simulink model "cart_pendulam"  (R2019a)
settings: Solver=VariableStepAuto  StartTime=0.0  StopTime=inf  FixedStep=0.01  MaxStep=0.05  MinStep=0.001  RelTol=1e-3
undefined symbols (not defined in the file): sigbuilder_block
settings Model: Creator=HPP  LastModifiedBy=vardhah
settings SolverCC: InitialStep=0.01
settings DebuggingCC: UnderSpecifiedDimensionMsg=warning

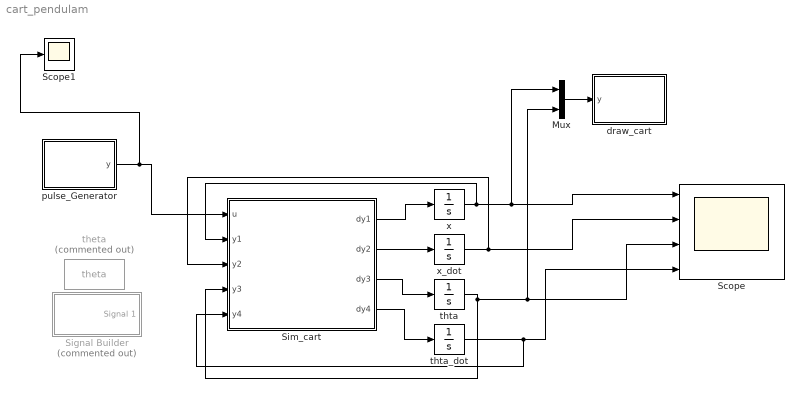
== system cart_pendulam ==
  Mux : Mux  Inputs=2
  Scope : Scope  NumInputPorts=4
  Scope1 : Scope
  Signal Builder : Subsystem  Tag=STV Subsys  Commented=on  LoadFcn=sigbuilder_block('load');  StartFcn=sigbuilder_block('start');  StopFcn=sigbuilder_block('stop');  ClipboardFcn=sigbuilder_block('clipboard');  mask(Sigbuilder block){tuvar=[0:10]}
      mask help: Simulink:masks:SigbuilderBlock_MD
      mask init:
      | if ~strcmp(get_param(bdroot(gcbh),'SimulationStatus'),'stopped') tuvar = sigbuilder_block('maskInit'); end
      settings: CopyFcn=sigbuilder_block('copy');  DeleteFcn=sigbuilder_block('delete');  ModelCloseFcn=sigbuilder_block('modelClose');  PreSaveFcn=sigbuilder_block('preSave');  PauseFcn=sigbuilder_block('pause');  ContinueFcn=sigbuilder_block('continue');  NameChangeFcn=sigbuilder_block('namechange');  OpenFcn=sigbuilder_block('open',[437.6 199.2 550.4 400 ]);  CloseFcn=sigbuilder_block('close');
      mask Display: plot(0, 0, 100, 100,[2, 2, 32, 32, 2], [68, 8, 8, 68, 68],[32, 2], [38, 38], [32, 19, 2],[53, 60, 44], [32, 17, 17, 2],[16, 16, 31, 31]);txt = getActiveGroup(gcbh);text(2, 100, txt,'verticalAlignment', 'top');
  Sim_cart : MATLAB Function  TreatAsAtomicUnit=on
  draw_cart : MATLAB Function  TreatAsAtomicUnit=on
  pulse_Generator : MATLAB Function  TreatAsAtomicUnit=on
  theta : ToWorkspace  Commented=on  VariableName=theta  SaveFormat=Timeseries  SampleTime=-1
  thta : Integrator
  thta_dot : Integrator
  x : Integrator
  x_dot : Integrator
  wires:
  Sim_cart/1(dy1) -> x/1
  Sim_cart/2(dy2) -> x_dot/1
  Sim_cart/3(dy3) -> thta/1
  Sim_cart/4(dy4) -> thta_dot/1
  x/1 -> Sim_cart/2(y1), Mux/1, Scope/1
  x_dot/1 -> Sim_cart/3(y2), Scope/2
  thta_dot/1 -> Sim_cart/5(y4), Scope/4
  pulse_Generator/1(y) -> Scope1/1, Sim_cart/1(u)
  thta/1 -> Sim_cart/4(y3), Mux/2, Scope/3
  Mux/1 -> draw_cart/1(y)

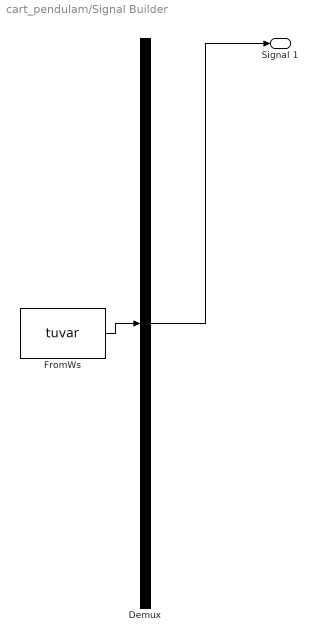
== system cart_pendulam/Signal Builder ==
  Demux : Demux  Tag=STV Demux  Outputs=1
  FromWs : FromWorkspace  Tag=STV FromWs  VariableName=tuvar  SampleTime=0
      SigBuilderData=|
      | common.afterFinalStr = 'Extrapolate'
      | common.sampleTime = 0
      | dataSet.timeRange = [0 10]
      | dataSet.name = 'Group 1'
      | sbobj.Groups.Name = 'Group 1'
      | sbobj.Groups.Signals.Name = 'Signal 1'
      | sbobj.Groups.Signals.XData = [0 4 4 6 6 10]
      | sbobj.Groups.Signals.YData = [0 0 1 1 0 0]
  Signal 1 : Outport  Tag=STV Outport
  wires:
  Demux/1 -> Signal 1/1
  FromWs/1 -> Demux/1

== matlab function cart_pendulam/draw_cart ==
  data: y input
function drawcartpend(y)
x = y(1);
th = y(2);

m = 1;
M = 5;
L = 2;
% kinematics
% x = 3;        % cart position
% th = 3*pi/2;   % pendulum angle

% dimensions
% L = 2;  % pendulum length
W = 1*sqrt(M/5);  % cart width
H = .5*sqrt(M/5); % cart height
wr = .2; % wheel radius
mr = .3*sqrt(m); % mass radius

% positions
% y = wr/2; % cart vertical position
y = wr/2+H/2; % cart vertical position
w1x = x-.9*W/2;
w1y = 0;
w2x = x+.9*W/2-wr;
w2y = 0;

px = x + L*sin(th);
py = y - L*cos(th);

plot([-10+x 10+x],[0 0],'k','LineWidth',2)
hold on
rectangle('Position',[x-W/2,y-H/2,W,H],'Curvature',.1,'FaceColor',[1 0.1 0.1])
rectangle('Position',[w1x,w1y,wr,wr],'Curvature',1,'FaceColor',[0 0 0])
rectangle('Position',[w2x,w2y,wr,wr],'Curvature',1,'FaceColor',[0 0 0])

plot([x px],[y py],'k','LineWidth',2)

rectangle('Position',[px-mr/2,py-mr/2,mr,mr],'Curvature',1,'FaceColor',[.1 0.1 1])

% set(gca,'YTick',[])
% set(gca,'XTick',[])
xlim([-10+x 10+x]);
ylim([-2 2.5]);
%set(gcf,'Position',[100 550 500 400])
% box off
drawnow
hold off

== matlab function cart_pendulam/Sim_cart ==
  settings: updateMethod=DISCRETE
  data: u input; y1 input; dy1 output size=1; dy2 output size=1; dy3 output size=1; dy4 output size=1; y2 input; y3 input; y4 input
function [dy1,dy2,dy3,dy4] = cartpend(u,y1,y2,y3,y4)

m = 1;
M = 5;
L = 2;
g = -10;
d = 1;

Sy = sin(y3);
Cy = cos(y3);
D = m*L*L*(M+m*(1-Cy^2));

dy1 = y2;
dy2 = (1/D)*(-m^2*L^2*g*Cy*Sy + m*L^2*(m*L*y4^2*Sy - d*y2)) + m*L*L*(1/D)*u;
dy3 = y4;
dy4 = (1/D)*((m+M)*m*g*L*Sy - m*L*Cy*(m*L*y4^2*Sy - d*y2)) - m*L*Cy*(1/D)*u ;
end

== matlab function cart_pendulam/pulse_Generator ==
  data: y output
function y = fcn()
persistent out;
persistent flag n calculate r;
persistent pulse_count pulse_size gap_count; 
sample_time=0.01;

%%
if isempty(r)
    r=1;
end

if isempty(calculate)
    calculate=0;
end
if isempty(pulse_count)
    pulse_count=uint32(0);
end
if isempty(pulse_size)
    pulse_size=0;
end
if isempty(gap_count)
    gap_count=uint32(0);
end
if isempty(out)
    out=0;
end
if isempty(flag)
    flag=1;
end
if isempty(n)
    n=0;
end
%%
if calculate==0 
 pulse_gap_duration=randn(1); 
 gap_count = uint32(pulse_gap_duration/sample_time); 
 pulse_size = 0.05+0.15*rand(1);
 pulse_count=uint32(pulse_size/sample_time);
 calculate=1;
 r = randi([-1 1], 1);
end
 n=n+1; 
 if n>gap_count && n<(gap_count+pulse_count)
     flag=0;
     out=r*1/pulse_size;   
 elseif n>(gap_count+pulse_count)
     flag=1;
     n=0;
     calculate=0;
 end

if flag==1
    out = 0; 
end
y = out;
